simulink model "UnitTestDebug"  (R2018b)
settings: Solver=FixedStepDiscrete  StartTime=0.0  StopTime=tfinal  FixedStep=fswParams.sample_time_s  RelTol=1e-3
undefined symbols (not defined in the file or in its folder): fswParams
libraries: aerolibutil x8, simulink x3, MEKF_lib x1, satelliteDynamics_lib x1
settings Model: SimulationMode=accelerator  Creator=satcave1  LastModifiedBy=kylle
settings OptimizationCC: EfficientMapNaN2IntZero=off
settings HardwareCC: TargetBitPerPointer=64  TargetBitPerSizeT=64  TargetBitPerPtrDiffT=64  TargetLongLongMode=on  TargetIntDivRoundTo=Zero  TargetEndianess=LittleEndian  TargetWordSize=64  TargetHWDeviceType=MATLAB Host  ProdEqTarget=off
settings CodeAppCC: MaxIdLength=128
settings GRTTargetCC: TargetLangStandard=C89/C90 (ANSI)  CombineOutputUpdateFcns=off  GRTInterface=on

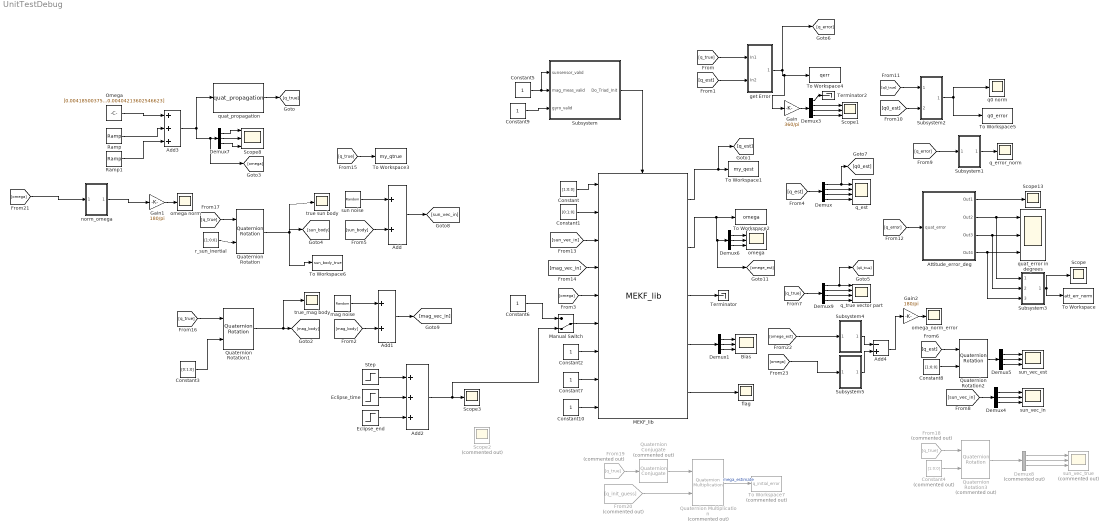
== system UnitTestDebug ==
  Add : Sum
  Add1 : Sum
  Add2 : Sum  Inputs=+++
  Add3 : Sum  Inputs=+++
  Add4 : Sum  Inputs=-+
  Attitude_error_deg : Subsystem
  Bias : Scope  NumInputPorts=3
  Constant : Constant  Value=[1;0;0]  VectorParams1D=off
  Constant1 : Constant  Value=[0;1;0]  VectorParams1D=off
  Constant{2,5..7,9..10} (6 alike) : Constant
  Constant3 : Constant  Value=[0;1;0]  VectorParams1D=off
  Constant4 : Constant  Commented=on  Value=[1;0;0]  VectorParams1D=off
  Constant8 : Constant  Value=[1;0;0]  VectorParams1D=off
  Demux : Demux
  Demux{1,4..7} (5 alike) : Demux  Outputs=3
  Demux3 : Demux
  Demux8 : Demux  Commented=on  Outputs=3
  Demux9 : Demux
  Eclipse_end : Step  Time=3700.0333  SampleTime=0
  Eclipse_time : Step  Time=1900  After=-1  SampleTime=0
  From18 : From  Commented=on  GotoTag=q_true
  From19 : From  Commented=on  GotoTag=q_true
  From20 : From  Commented=on  GotoTag=q_init_guess
  Gain : Gain  Gain=360/pi
  Gain1 : Gain  Gain=180/pi
  Gain2 : Gain  Gain=180/pi
  MEKF_lib : MEKF_lib/MEKF_lib  SystemSampleTime=-1
      link override Unit Delay: InitialCondition=fswParams.estimation.ic.Pchol_init
      link override Unit Delay2: InitialCondition=[0;0.707106781186547;0.707106781186547;0]
  Manual Switch : ManualSwitch  CurrentSetting=0
  Omega : Constant  Value=[0.00418500375565425;0.00650393994925115;0.00404213602546623]  VectorParams1D=off
  Quaternion Conjugate : aerolibutil/Quaternion Conjugate  Commented=on
      settings: SourceProductName=Aerospace Blockset  SourceProductBaseCode=AE
  Quaternion Multiplication : aerolibutil/Quaternion Multiplication  Commented=on
  Quaternion Rotation : aerolibutil/Quaternion Rotation
  Quaternion Rotation1 : aerolibutil/Quaternion Rotation
  Quaternion Rotation2 : aerolibutil/Quaternion Rotation
  Quaternion Rotation3 : aerolibutil/Quaternion Rotation  Commented=on
  Ramp : simulink/Sources/Ramp  slope=0.0008  start=0  InitialOutput=0
  Ramp1 : simulink/Sources/Ramp  slope=-0.0008  start=200  InitialOutput=0
  Scope : Scope
  Scope1 : Scope  NumInputPorts=3
  Scope13 : Scope
  Scope2 : Scope  Commented=on
  Scope3 : Scope
  Scope8 : Scope  NumInputPorts=3
  Step : Step  Time=0  SampleTime=0
  Subsystem : Subsystem
  Subsystem1 : Subsystem
  Subsystem2 : Subsystem
  Subsystem3 : Subsystem
  Subsystem4 : Subsystem
  Subsystem5 : Subsystem
  Terminator : Terminator
  Terminator2 : Terminator
  To Workspace : ToWorkspace  VariableName=att_err_norm  SaveFormat=Timeseries  SampleTime=-1
  To Workspace1 : ToWorkspace  VariableName=my_qest  SaveFormat=Timeseries  SampleTime=-1
  To Workspace2 : ToWorkspace  VariableName=omega  SaveFormat=Timeseries  SampleTime=-1
  To Workspace3 : ToWorkspace  VariableName=my_qtrue  SaveFormat=Timeseries  SampleTime=-1
  To Workspace4 : ToWorkspace  VariableName=qerr  SaveFormat=Timeseries  SampleTime=-1
  To Workspace5 : ToWorkspace  VariableName=q0_error  SaveFormat=Timeseries  SampleTime=-1
  To Workspace6 : ToWorkspace  VariableName=sun_body_true  SaveFormat=Timeseries  SampleTime=-1
  To Workspace7 : ToWorkspace  Commented=on  VariableName=q_initial_error  SaveFormat=Timeseries  SampleTime=-1
  flag : Scope
  get Error : Subsystem
  mag noise : RandomNumber  Variance=[2e-7;2e-7;2e-7];  SampleTime=fswParams.sample_time_s  VectorParams1D=off
  norm_omega : Subsystem
  omega : Scope  NumInputPorts=3
  omega norm : Scope
  omega_norm_error : Scope
  q0 norm : Scope
  q_error_norm : Scope
  q_est : Scope  NumInputPorts=4
  q_true vector part : Scope  NumInputPorts=4
  quat_error in degrees : Scope  NumInputPorts=3
  quat_propagation : satelliteDynamics_lib/satelliteDynamics_lib/quat_propagation  SystemSampleTime=-1
      link override Discrete-Time Integrator: InitialCondition=[0;0.707106781186547;0.707106781186547;0]
  r_sun_inertial : Constant  Value=[1;0;0]  VectorParams1D=off
  sun noise : RandomNumber  Variance=[6e-4;6e-4;6e-4];  SampleTime=fswParams.sample_time_s  VectorParams1D=off
  sun_vec_est : Scope  NumInputPorts=3
  sun_vec_in : Scope  NumInputPorts=3
  sun_vec_true : Scope  Commented=on  NumInputPorts=3
  true sun body : Scope
  true_mag body : Scope
  wires:
  Quaternion Rotation/1 -> To Workspace6/1, true sun body/1, [sun_body]
  Demux/2 -> q_est/2
  Demux/3 -> q_est/3
  Demux/4 -> q_est/4
  Demux1/2 -> Bias/2
  Demux1/1 -> Bias/1
  Demux1/3 -> Bias/3
  r_sun_inertial/1 -> Quaternion Rotation/2
  Constant3/1 -> Quaternion Rotation1/2
  quat_propagation/1 -> [q_true]
  Quaternion Rotation1/1 -> [mag_body], true_mag body/1
  Constant7/1 -> MEKF_lib/8
  Constant/1 -> MEKF_lib/1
  Constant1/1 -> MEKF_lib/2
  MEKF_lib/3 -> Terminator/1
  MEKF_lib/4 -> Demux1/1
  MEKF_lib/1 -> [q_est], To Workspace1/1
  [omega] -> MEKF_lib/5
  [sun_body] -> Add/2
  sun noise/1 -> Add/1
  mag noise/1 -> Add1/1
  [mag_body] -> Add1/2
  Demux4/1 -> sun_vec_in/1
  Demux4/3 -> sun_vec_in/3
  Demux4/2 -> sun_vec_in/2
  Add/1 -> [sun_vec_in]
  Constant8/1 -> Quaternion Rotation2/2
  [q_est] -> Quaternion Rotation2/1
  Quaternion Rotation2/1 -> Demux5/1
  Demux5/1 -> sun_vec_est/1
  Demux5/2 -> sun_vec_est/2
  Demux6/2 -> omega/2
  Demux6/1 -> omega/1
  Demux6/3 -> omega/3
  MEKF_lib/2 -> [omege_est], Demux6/1, To Workspace2/1
  Constant10/1 -> MEKF_lib/9
  MEKF_lib/5 -> flag/1
  Demux7/1 -> Scope8/1
  Omega/1 -> Add3/1
  Demux7/2 -> Scope8/2
  Demux7/3 -> Scope8/3
  Constant9/1 -> Subsystem/3(gyro_valid)
  Subsystem/1(Do_Triad_Init) -> MEKF_lib/Enable
  Constant5/1 -> Subsystem/1(sunsensor_valid), Subsystem/2(mag_meas_valid)
  Demux5/3 -> sun_vec_est/3
  Attitude_error_deg/1(Out1) -> Scope13/1
  Attitude_error_deg/2(Out2) -> Subsystem3/1(In1), quat_error in degrees/1
  Attitude_error_deg/4(Out4) -> Subsystem3/3(In3), quat_error in degrees/3
  [q_true] -> Demux9/1
  [q_error] -> Subsystem1/1(In1)
  Subsystem1/1(Out1) -> q_error_norm/1
  Subsystem2/1(Out1) -> To Workspace5/1, q0 norm/1
  [q0_true] -> Subsystem2/1(In1)
  [q0_est] -> Subsystem2/2(In2)
  [q_true] -> get Error/1(In1)
  [q_est] -> get Error/2(In2)
  [q_error] -> Attitude_error_deg/1(quat_error)
  [sun_vec_in] -> Demux4/1
  [sun_vec_in] -> MEKF_lib/3
  [mag_vec_in] -> MEKF_lib/4
  Add1/1 -> [mag_vec_in]
  [q_true] -> To Workspace3/1
  [q_true] -> Quaternion Rotation1/1
  [q_true] -> Quaternion Rotation/1
  [q_est] -> Demux/1
  Demux/1 -> [q0_est], q_est/1
  Demux9/4 -> q_true vector part/4
  Demux9/3 -> q_true vector part/3
  Demux9/2 -> q_true vector part/2
  Demux9/1 -> [q0_true], q_true vector part/1
  Attitude_error_deg/3(Out3) -> Subsystem3/2(In2), quat_error in degrees/2
  Subsystem3/1(Out1) -> Scope/1, To Workspace/1
  get Error/1(mega_estimate) -> To Workspace4/1, Gain/1, [q_error]
  Demux3/3 -> Scope1/2
  Demux3/4 -> Scope1/3
  Demux3/1 -> Terminator2/1
  Demux3/2 -> Scope1/1
  Gain/1 -> Demux3/1
  Demux8/1 -> sun_vec_true/1
  From18/1 -> Quaternion Rotation3/1
  Constant4/1 -> Quaternion Rotation3/2
  Demux8/2 -> sun_vec_true/2
  Quaternion Rotation3/1 -> Demux8/1
  Demux8/3 -> sun_vec_true/3
  From20/1 -> Quaternion Multiplication/2
  Quaternion Conjugate/1 -> Quaternion Multiplication/1
  From19/1 -> Quaternion Conjugate/1
  Quaternion Multiplication/1 -> To Workspace7/1  "mega_estimate"
  Step/1 -> Add2/1
  Eclipse_time/1 -> Add2/2
  Add2/1 -> Manual Switch/2, Scope3/1
  Constant2/1 -> MEKF_lib/7
  Eclipse_end/1 -> Add2/3
  Manual Switch/1 -> MEKF_lib/6
  Constant6/1 -> Manual Switch/1
  Add3/1 -> quat_propagation/1, [omega], Demux7/1
  Ramp/1 -> Add3/2
  Ramp1/1 -> Add3/3
  Gain1/1 -> omega norm/1
  [omege_est] -> Subsystem4/1(In1)
  [omega] -> Subsystem5/1(In1)
  [omega] -> norm_omega/1(In1)
  norm_omega/1(Out1) -> Gain1/1
  Subsystem4/1(Out1) -> Add4/1
  Subsystem5/1(Out1) -> Add4/2
  Gain2/1 -> omega_norm_error/1
  Add4/1 -> Gain2/1

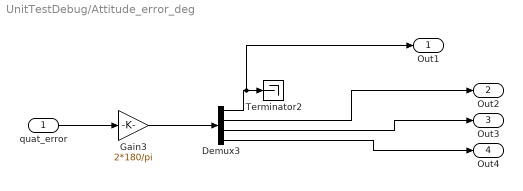
== system UnitTestDebug/Attitude_error_deg ==
  quat_error : Inport
  Demux3 : Demux
  Gain3 : Gain  Gain=2*180/pi
  Terminator2 : Terminator
  Out1 : Outport
  Out2 : Outport  Port=2
  Out3 : Outport  Port=3
  Out4 : Outport  Port=4
  wires:
  Demux3/2 -> Out2/1
  quat_error/1 -> Gain3/1
  Demux3/1 -> Out1/1, Terminator2/1
  Demux3/4 -> Out4/1
  Demux3/3 -> Out3/1
  Gain3/1 -> Demux3/1

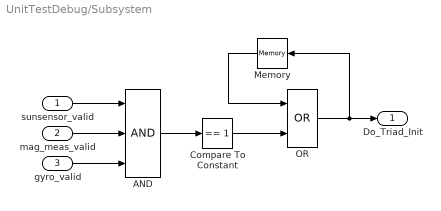
== system UnitTestDebug/Subsystem ==
  sunsensor_valid : Inport
  mag_meas_valid : Inport  Port=2
  gyro_valid : Inport  Port=3
  AND : Logic  Inputs=3  IconShape=distinctive  AllPortsSameDT=off  OutDataTypeStr=boolean
  Compare To Constant : simulink/Logic and Bit Operations/Compare To Constant  relop===  const=1  OutDataTypeStr=boolean
  Memory : Memory
  OR : Logic  Operator=OR  AllPortsSameDT=off  OutDataTypeStr=boolean
  Do_Triad_Init : Outport
  wires:
  mag_meas_valid/1 -> AND/2
  Compare To Constant/1 -> OR/2
  OR/1 -> Do_Triad_Init/1, Memory/1
  Memory/1 -> OR/1
  AND/1 -> Compare To Constant/1
  sunsensor_valid/1 -> AND/1
  gyro_valid/1 -> AND/3

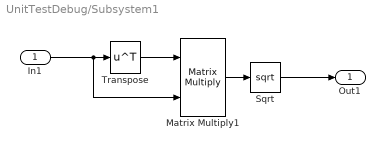
== system UnitTestDebug/Subsystem1 ==
  In1 : Inport
  Matrix Multiply1 : Product  Multiplication=Matrix(*)
  Sqrt : Sqrt  SaturateOnIntegerOverflow=on
  Transpose : Math  Operator=transpose  SaturateOnIntegerOverflow=on
  Out1 : Outport
  wires:
  In1/1 -> Matrix Multiply1/2, Transpose/1
  Matrix Multiply1/1 -> Sqrt/1
  Transpose/1 -> Matrix Multiply1/1
  Sqrt/1 -> Out1/1

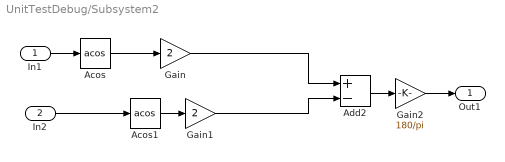
== system UnitTestDebug/Subsystem2 ==
  In1 : Inport
  In2 : Inport  Port=2
  Acos : Trigonometry  Operator=acos
  Acos1 : Trigonometry  Operator=acos
  Add2 : Sum  Inputs=+-
  Gain : Gain  Gain=2
  Gain1 : Gain  Gain=2
  Gain2 : Gain  Gain=180/pi
  Out1 : Outport
  wires:
  Gain1/1 -> Add2/2
  Acos/1 -> Gain/1
  Gain/1 -> Add2/1
  Acos1/1 -> Gain1/1
  Add2/1 -> Gain2/1
  In1/1 -> Acos/1
  In2/1 -> Acos1/1
  Gain2/1 -> Out1/1

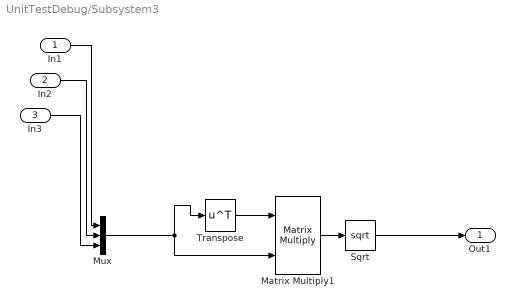
== system UnitTestDebug/Subsystem3 ==
  In1 : Inport
  In2 : Inport  Port=2
  In3 : Inport  Port=3
  Matrix Multiply1 : Product  Multiplication=Matrix(*)
  Mux : Mux  Inputs=3
  Sqrt : Sqrt  SaturateOnIntegerOverflow=on
  Transpose : Math  Operator=transpose  SaturateOnIntegerOverflow=on
  Out1 : Outport
  wires:
  Mux/1 -> Transpose/1, Matrix Multiply1/2
  In3/1 -> Mux/3
  Sqrt/1 -> Out1/1
  Matrix Multiply1/1 -> Sqrt/1
  Transpose/1 -> Matrix Multiply1/1
  In2/1 -> Mux/2
  In1/1 -> Mux/1

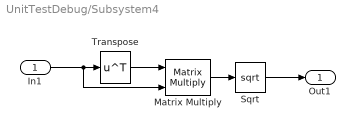
== system UnitTestDebug/Subsystem4 ==
  In1 : Inport
  Matrix Multiply : Product  Multiplication=Matrix(*)
  Sqrt : Sqrt  SaturateOnIntegerOverflow=on
  Transpose : Math  Operator=transpose  SaturateOnIntegerOverflow=on
  Out1 : Outport
  wires:
  In1/1 -> Matrix Multiply/2, Transpose/1
  Transpose/1 -> Matrix Multiply/1
  Matrix Multiply/1 -> Sqrt/1
  Sqrt/1 -> Out1/1

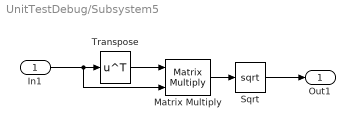
== system UnitTestDebug/Subsystem5 ==
  In1 : Inport
  Matrix Multiply : Product  Multiplication=Matrix(*)
  Sqrt : Sqrt  SaturateOnIntegerOverflow=on
  Transpose : Math  Operator=transpose  SaturateOnIntegerOverflow=on
  Out1 : Outport
  wires:
  In1/1 -> Matrix Multiply/2, Transpose/1
  Transpose/1 -> Matrix Multiply/1
  Matrix Multiply/1 -> Sqrt/1
  Sqrt/1 -> Out1/1

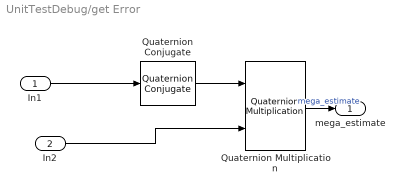
== system UnitTestDebug/get Error ==
  In1 : Inport
  In2 : Inport  Port=2
  Quaternion Conjugate : aerolibutil/Quaternion Conjugate
      settings: SourceProductName=Aerospace Blockset  SourceProductBaseCode=AE
  Quaternion Multiplication : aerolibutil/Quaternion Multiplication
  mega_estimate : Outport
  wires:
  Quaternion Conjugate/1 -> Quaternion Multiplication/1
  Quaternion Multiplication/1 -> mega_estimate/1  "mega_estimate"
  In1/1 -> Quaternion Conjugate/1
  In2/1 -> Quaternion Multiplication/2

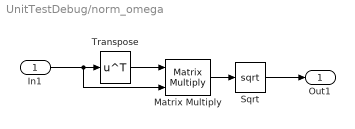
== system UnitTestDebug/norm_omega ==
  In1 : Inport
  Matrix Multiply : Product  Multiplication=Matrix(*)
  Sqrt : Sqrt  SaturateOnIntegerOverflow=on
  Transpose : Math  Operator=transpose  SaturateOnIntegerOverflow=on
  Out1 : Outport
  wires:
  In1/1 -> Matrix Multiply/2, Transpose/1
  Transpose/1 -> Matrix Multiply/1
  Matrix Multiply/1 -> Sqrt/1
  Sqrt/1 -> Out1/1
